simulink model "plant_control_full"  (R2023a)
settings: Solver=FixedStepAuto  StartTime=0.0  StopTime=10.0  FixedStep=0.01  RelTol=1e-3
values from neighbouring files (symbols this model uses):
  g = 9.81    [full_loop.m]    (also in inner_loop.m)
  KI = K(:,1:2)    [LQR_PI.m]    (also in full_loop.m = K(:,1:nref); inner_loop.m = K(:,1:3))
  Kp_x = K(:,3:5)    [LQR_PI.m]    (also in full_loop.m = K(:,nref+1:np+nref); inner_loop.m = K(:,4:9))
  Kp_xref = K(:,6:7)    [LQR_PI.m]    (also in full_loop.m = K(:,np+nref+1:end); inner_loop.m = K(:,10:12))
  m = 10    [full_loop.m]    (also in inner_loop.m)
  sys_p = ss(Ap, Bp, Cp, Dp)    [LQR_PI.m]    (also in full_loop.m = ss(Ap, Bp, Cp([1:3,9],:), zeros(nref, mp)); inner_loop.m = ss(Ap(1:np, 1:np), Bp(1:np, :), Cp(:, 1:np), Dp))
  sys_ref = ss(A_ref, B_ref, C_ref, D_ref)    [LQR_PI.m]    (also in full_loop.m; inner_loop.m)
libraries: simulink_extras x1, shared6dof x1
settings Model: Creator=timme  LastModifiedBy=timme
settings OptimizationCC: BlockReduction=off  DefaultParameterBehavior=Inlined  BufferReuse=off

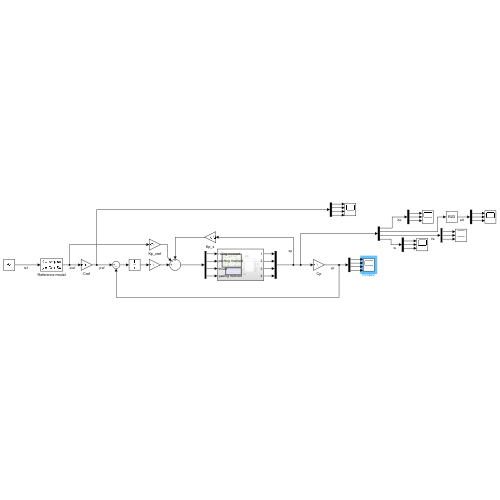
[thumbnail: Simulink's stored preview of the top-level diagram]
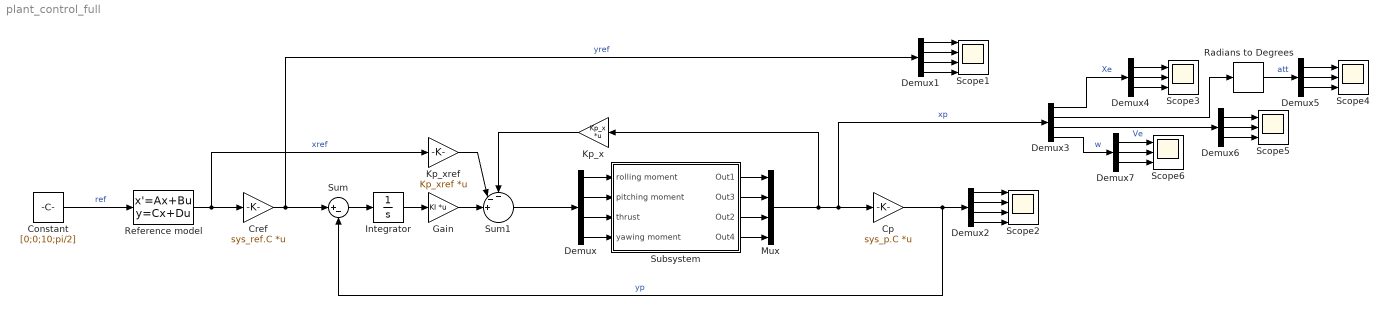
== system plant_control_full ==
  Constant : Constant  Value=[0;0;10;pi/2]
  Cp : Gain  Gain=sys_p.C  Multiplication=Matrix(K*u)
  Cref : Gain  Gain=sys_ref.C  Multiplication=Matrix(K*u)
  Demux : Demux
  Demux1 : Demux
  Demux2 : Demux
  Demux3 : Demux  Outputs=[3 3 3 3]
  Demux{4..7} (4 alike) : Demux  Outputs=3
  Gain : Gain  Gain=KI  Multiplication=Matrix(K*u)
  Integrator : Integrator
  Kp_x : Gain  Gain=Kp_x  Multiplication=Matrix(K*u)
  Kp_xref : Gain  Gain=Kp_xref  Multiplication=Matrix(K*u)
  Mux : Mux
  Radians to Degrees : simulink_extras/Transformations/Radians to Degrees
  Reference model : StateSpace  A=sys_ref.A  B=sys_ref.B  C=sys_ref.C  D=sys_ref.D  InitialCondition=0
  Scope1 : Scope  NumInputPorts=4
  Scope2 : Scope  NumInputPorts=4
  Scope{3..6} (4 alike) : Scope  NumInputPorts=3
  Subsystem : Subsystem
  Sum : Sum  Inputs=|+-
  Sum1 : Sum  Inputs=--+||
  wires:
  Mux/1 -> Demux3/1, Cp/1, Kp_x/1  "xp"
  Cp/1 -> Demux2/1, Sum/2  "yp"
  Sum/1 -> Integrator/1
  Integrator/1 -> Gain/1
  Gain/1 -> Sum1/3
  Sum1/1 -> Demux/1
  Reference model/1 -> Kp_xref/1, Cref/1  "xref"
  Cref/1 -> Demux1/1, Sum/1  "yref"
  Constant/1 -> Reference model/1  "ref"
  Kp_xref/1 -> Sum1/2
  Kp_x/1 -> Sum1/1
  Demux1/3 -> Scope1/3
  Demux1/2 -> Scope1/2
  Demux1/1 -> Scope1/1
  Demux1/4 -> Scope1/4
  Demux2/3 -> Scope2/3
  Demux2/4 -> Scope2/4
  Demux2/2 -> Scope2/2
  Demux2/1 -> Scope2/1
  Demux/1 -> Subsystem/1(rolling moment)
  Demux/2 -> Subsystem/2(pitching moment)
  Demux/3 -> Subsystem/3(thrust)
  Demux/4 -> Subsystem/4(yawing moment)
  Subsystem/1(Out1) -> Mux/1
  Subsystem/4(Out4) -> Mux/4
  Subsystem/2(Out3) -> Mux/2
  Subsystem/3(Out2) -> Mux/3
  Demux4/2 -> Scope3/2
  Demux4/3 -> Scope3/3
  Demux4/1 -> Scope3/1
  Demux3/1 -> Demux4/1  "Xe"
  Demux3/2 -> Radians to Degrees/1
  Demux5/3 -> Scope4/3
  Demux5/1 -> Scope4/1
  Demux5/2 -> Scope4/2
  Demux6/2 -> Scope5/2
  Demux6/1 -> Scope5/1
  Demux6/3 -> Scope5/3
  Demux3/3 -> Demux6/1  "Ve"
  Demux7/2 -> Scope6/2
  Demux7/3 -> Scope6/3
  Demux3/4 -> Demux7/1  "w"
  Demux7/1 -> Scope6/1
  Radians to Degrees/1 -> Demux5/1  "att"

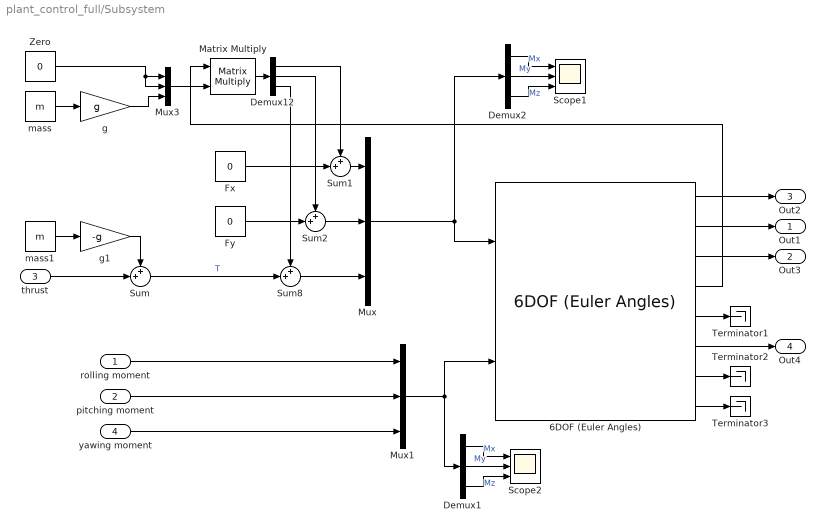
== system plant_control_full/Subsystem ==
  rolling moment : Inport
  pitching moment : Inport  Port=2
  thrust : Inport  Port=3
  yawing moment : Inport  Port=4
  6DOF (Euler Angles) : shared6dof/6DOF (Euler Angles)  units=Metric (MKS)  mtype=Fixed  rep=Euler Angles  xme_0=[0 0 0]  Vm_0=[0 0 0]  eul_0=[0 0 0]  pm_0=[0 0 0]  mass_0=m  mass_e=0.5  mass_f=2.0  inertia=I  inertia_e=eye(3)  inertia_f=2*eye(3)  k_quat=1.0  vre_flag=on  abi_flag=off  aMode=0  xme_statename=''  Vm_statename=''  eul_statename=''  quat_statename=''  pm_statename=''  mass_statename=''
  Demux1 : Demux  Outputs=3
  Demux12 : Demux  Outputs=3
  Demux2 : Demux  Outputs=3
  Fx : Constant  Value=0
  Fy : Constant  Value=0
  Matrix Multiply : Product  Inputs=**  Multiplication=Matrix(*)
  Mux : Mux  Inputs=3
  Mux1 : Mux  Inputs=3
  Mux3 : Mux  Inputs=3
  Scope1 : Scope  NumInputPorts=3
  Scope2 : Scope  NumInputPorts=3
  Sum{,1..2,8} (4 alike) : Sum  Inputs=++|
  Terminator1 : Terminator
  Terminator2 : Terminator
  Terminator3 : Terminator
  Zero : Constant  Value=0  OutDataTypeStr=Inherit: Inherit via back propagation
  g : Gain  Gain=g
  g1 : Gain  Gain=-g
  mass : Constant  Value=m
  mass1 : Constant  Value=m
  Out1 : Outport
  Out3 : Outport  Port=2
  Out2 : Outport  Port=3
  Out4 : Outport  Port=4
  wires:
  6DOF (Euler Angles)/1 -> Out2/1
  Demux12/2 -> Sum2/1
  Demux12/1 -> Sum1/1
  Demux1/3 -> Scope2/3  "Mz"
  rolling moment/1 -> Mux1/1
  6DOF (Euler Angles)/8 -> Terminator3/1
  6DOF (Euler Angles)/2 -> Out1/1
  Demux2/3 -> Scope1/3  "Mz"
  6DOF (Euler Angles)/7 -> Terminator2/1
  thrust/1 -> Sum/2
  pitching moment/1 -> Mux1/2
  Mux1/1 -> 6DOF (Euler Angles)/2, Demux1/1
  g/1 -> Mux3/3
  Zero/1 -> Mux3/1, Mux3/2
  Sum2/1 -> Mux/2
  6DOF (Euler Angles)/6 -> Out4/1
  Demux1/1 -> Scope2/1  "Mx"
  mass/1 -> g/1
  yawing moment/1 -> Mux1/3
  Matrix Multiply/1 -> Demux12/1
  Mux/1 -> Demux2/1, 6DOF (Euler Angles)/1
  6DOF (Euler Angles)/5 -> Terminator1/1
  Sum8/1 -> Mux/3
  Demux2/1 -> Scope1/1  "Mx"
  Sum/1 -> Sum8/2  "T"
  6DOF (Euler Angles)/4 -> Matrix Multiply/1
  Sum1/1 -> Mux/1
  Demux12/3 -> Sum8/1
  6DOF (Euler Angles)/3 -> Out3/1
  Fy/1 -> Sum2/2
  g1/1 -> Sum/1
  Fx/1 -> Sum1/2
  Demux1/2 -> Scope2/2  "My"
  Mux3/1 -> Matrix Multiply/2
  mass1/1 -> g1/1
  Demux2/2 -> Scope1/2  "My"
